simulink model "uz_mlp_three_layer"  (R2021a)
settings: Solver=FixedStepDiscrete  StartTime=0.0  StopTime=5000  RelTol=1e-3
values from neighbouring files (symbols this model uses):
  nn = nn.set_all_parameter(rand_variables)    [mlp2_definition.m]
  nn_data_type_max = 131071    [mlp2_definition.m]
  numInput = 13    [mlp2_definition.m]
  numOut = 4    [mlp2_definition.m]
libraries: hdlsllib x90, simulink x79, el_machinelearning x2
(part 1 of 4)
settings Model: DataTypeOverride=Off  Creator=ts  LastModifiedBy=ts
settings SolverCC: AlgebraicLoopSolver=TrustRegion
settings DataIOCC: SaveOutput=off  SaveTime=off
settings OptimizationCC: BlockReduction=off  ConditionallyExecuteInputs=off  DefaultParameterBehavior=Inlined
settings DebuggingCC: AlgebraicLoopMsg=error  SingleTaskRateTransMsg=error  SFMachineParentedDataDiag=warning
settings HardwareCC: ProdBitPerPointer=32  ProdBitPerSizeT=32  ProdBitPerPtrDiffT=32  ProdLargestAtomicFloat=None  ProdIntDivRoundTo=Undefined  ProdEndianess=Unspecified  ProdWordSize=32  ProdHWDeviceType=ASIC/FPGA->ASIC/FPGA  TargetBitPerLong=64  TargetBitPerPointer=64  TargetBitPerSizeT=64  TargetBitPerPtrDiffT=64  TargetLongLongMode=on  TargetIntDivRoundTo=Zero  TargetEndianess=LittleEndian  TargetWordSize=64  TargetHWDeviceType=Custom Processor->MATLAB Host Computer  ProdEqTarget=off

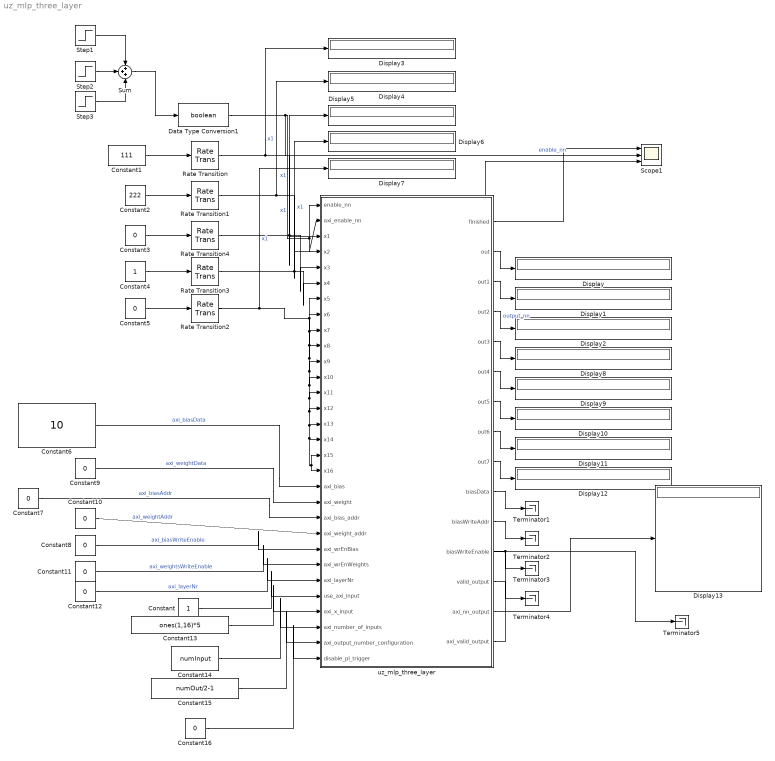
== system uz_mlp_three_layer ==
  Constant : Constant  OutDataTypeStr=boolean  SampleTime=-1
  Constant1 : Constant  Value=111  OutDataTypeStr=fixdt(1,32,14)
  Constant10 : Constant  Value=0  OutDataTypeStr=fixdt(0,10,0)  SampleTime=-1
  Constant11 : Constant  Value=0  OutDataTypeStr=uint8  SampleTime=-1
  Constant12 : Constant  Value=0  OutDataTypeStr=uint8  SampleTime=-1
  Constant13 : Constant  Value=ones(1,16)*5  OutDataTypeStr=fixdt(1,32,14)  SampleTime=-1
  Constant14 : Constant  Value=numInput  OutDataTypeStr=fixdt(0,10,0)  SampleTime=-1
  Constant15 : Constant  Value=numOut/2-1  OutDataTypeStr=fixdt(0,10,0)  SampleTime=-1
  Constant16 : Constant  Value=0  OutDataTypeStr=boolean  SampleTime=-1
  Constant2 : Constant  Value=222  OutDataTypeStr=fixdt(1,32,14)
  Constant3 : Constant  Value=0  OutDataTypeStr=fixdt(1,32,14)
  Constant4 : Constant  OutDataTypeStr=fixdt(1,32,14)
  Constant5 : Constant  Value=0  OutDataTypeStr=fixdt(1,32,14)
  Constant6 : Constant  Value=10  OutDataTypeStr=fixdt(1,32,14)  SampleTime=-1
  Constant7 : Constant  Value=0  OutDataTypeStr=fixdt(0,10,0)  SampleTime=-1
  Constant8 : Constant  Value=0  OutDataTypeStr=uint8  SampleTime=-1
  Constant9 : Constant  Value=0  OutDataTypeStr=fixdt(1,32,14)  SampleTime=-1
  Data Type Conversion1 : DataTypeConversion  OutDataTypeStr=boolean
  Display{,1..13} (14 alike) : Display
      Display11 settings: Format=hex (Stored Integer)
      Display3 settings: Format=hex (Stored Integer)
      Display4 settings: Format=hex (Stored Integer)
      Display5 settings: Format=hex (Stored Integer)
      Display6 settings: Format=hex (Stored Integer)
      Display7 settings: Format=hex (Stored Integer)
  Rate Transition{,1..4} (5 alike) : RateTransition
  Scope1 : Scope  NumInputPorts=3
  Step1 : Step  Time=2000  After=-1  SampleTime=1
  Step2 : Step  Time=100  SampleTime=1
  Step3 : Step  Time=2500  SampleTime=1
  Sum : Sum  Inputs=+++
  Terminator{1..5} (5 alike) : Terminator
  uz_mlp_three_layer : Subsystem  TreatAsAtomicUnit=on
  wires:
  Constant1/1 -> Rate Transition/1
  Constant5/1 -> Rate Transition2/1
  Constant2/1 -> Rate Transition1/1
  Constant3/1 -> Rate Transition4/1
  Constant4/1 -> Rate Transition3/1
  Data Type Conversion1/1 -> Scope1/2, uz_mlp_three_layer/2(axi_enable_nn), uz_mlp_three_layer/1(enable_nn)  "enable_nn"
  Rate Transition/1 -> uz_mlp_three_layer/3(x1), Display3/1  "x1"
  Rate Transition1/1 -> uz_mlp_three_layer/4(x2), Display4/1  "x1"
  Rate Transition4/1 -> Display5/1, uz_mlp_three_layer/5(x3)  "x1"
  Rate Transition3/1 -> Display6/1, uz_mlp_three_layer/6(x4)  "x1"
  Rate Transition2/1 -> uz_mlp_three_layer/8(x6), uz_mlp_three_layer/18(x16), uz_mlp_three_layer/17(x15), uz_mlp_three_layer/16(x14), uz_mlp_three_layer/15(x13), uz_mlp_three_layer/14(x12), uz_mlp_three_layer/13(x11), uz_mlp_three_layer/12(x10), uz_mlp_three_layer/11(x9), uz_mlp_three_layer/10(x8), uz_mlp_three_layer/9(x7), uz_mlp_three_layer/7(x5), Display7/1  "x1"
  uz_mlp_three_layer/2(out) -> Display/1
  uz_mlp_three_layer/3(out1) -> Display1/1
  uz_mlp_three_layer/4(out2) -> Display2/1  "output_nn"
  uz_mlp_three_layer/5(out3) -> Display8/1
  uz_mlp_three_layer/6(out4) -> Display9/1
  uz_mlp_three_layer/7(out5) -> Display10/1
  uz_mlp_three_layer/8(out6) -> Display11/1
  uz_mlp_three_layer/9(out7) -> Display12/1
  Constant6/1 -> uz_mlp_three_layer/19(axi_bias)  "axi_biasData"
  Constant7/1 -> uz_mlp_three_layer/21(axi_bias_addr)  "axi_biasAddr"
  Constant9/1 -> uz_mlp_three_layer/20(axi_weight)  "axi_weightData"
  Constant10/1 -> uz_mlp_three_layer/22(axi_weight_addr)  "axi_weightAddr"
  Constant8/1 -> uz_mlp_three_layer/23(axi_wrEnBias)  "axi_biasWriteEnable"
  Constant11/1 -> uz_mlp_three_layer/24(axi_wrEnWeights)  "axi_weightsWriteEnable"
  Constant12/1 -> uz_mlp_three_layer/25(axi_layerNr)  "axi_layerNr"
  uz_mlp_three_layer/10(biasData) -> Terminator1/1
  uz_mlp_three_layer/11(biasWriteAddr) -> Terminator2/1
  uz_mlp_three_layer/12(biasWriteEnable) -> Terminator3/1
  Step1/1 -> Sum/1
  Sum/1 -> Data Type Conversion1/1
  Step2/1 -> Sum/2
  Step3/1 -> Sum/3
  uz_mlp_three_layer/13(valid_output) -> Terminator4/1
  Constant/1 -> uz_mlp_three_layer/26(use_axi_input)
  Constant13/1 -> uz_mlp_three_layer/27(axi_x_input)
  uz_mlp_three_layer/14(axi_nn_output) -> Display13/1
  uz_mlp_three_layer/15(axi_valid_output) -> Scope1/3, Terminator5/1
  Constant14/1 -> uz_mlp_three_layer/28(axi_number_of_inputs)
  Constant15/1 -> uz_mlp_three_layer/29(axi_output_number_configuration)
  uz_mlp_three_layer/1(finished) -> Scope1/1
  Constant16/1 -> uz_mlp_three_layer/30(disable_pl_trigger)

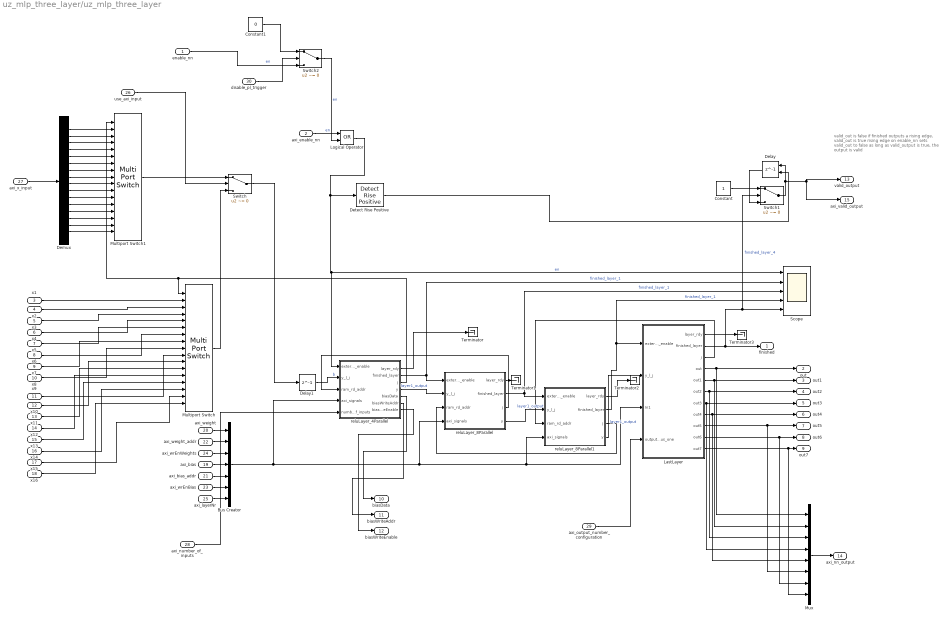
== system uz_mlp_three_layer/uz_mlp_three_layer ==
  note: valid_out is false
      | if finished outputs a rising edge, valid_out is true
      | rising edge on enable_nn sets valid_out to false
      |
      | as long as valid_output is true, the output is valid
  enable_nn : Inport
  axi_enable_nn : Inport  Port=2
  x1 : Inport  Port=3
  x2 : Inport  Port=4
  x3 : Inport  Port=5
  x4 : Inport  Port=6
  x5 : Inport  Port=7
  x6 : Inport  Port=8
  x7 : Inport  Port=9
  x8 : Inport  Port=10
  x9 : Inport  Port=11
  x10 : Inport  Port=12
  x11 : Inport  Port=13
  x12 : Inport  Port=14
  x13 : Inport  Port=15
  x14 : Inport  Port=16
  x15 : Inport  Port=17
  x16 : Inport  Port=18
  axi_bias : Inport  Port=19
  axi_weight : Inport  Port=20
  axi_bias_addr : Inport  Port=21
  axi_weight_addr : Inport  Port=22
  axi_wrEnBias : Inport  Port=23
  axi_wrEnWeights : Inport  Port=24
  axi_layerNr : Inport  Port=25
  use_axi_input : Inport  Port=26
  axi_x_input : Inport  Port=27
  axi_number_of_inputs : Inport  Port=28
  axi_output_number_configuration : Inport  Port=29
  disable_pl_trigger : Inport  Port=30
  Bus Creator : BusCreator  Inputs=7
  Constant : Constant  OutDataTypeStr=boolean  SampleTime=-1
  Constant1 : Constant  Value=0  OutDataTypeStr=boolean  SampleTime=-1
  Delay : Delay  DelayLength=1  ExternalReset=Level
      settings: InputPortMap=u0,r5
  Delay1 : Delay  DelayLength=1
  Demux : Demux  Outputs=16
  Detect Rise Positive : simulink/Logic and Bit Operations/Detect Rise Positive  vinit=0  OutDataTypeStr=boolean
  LastLayer : Subsystem  TreatAsAtomicUnit=on  mask{layer=nn.layer(4), ParallelDSP=2, nNeurons=numOut, LayerNr=4}
      mask prompts: layer "Layer number:"; ParallelDSP "Number of parallel DSP"; nNeurons "Number of neurons in layer"; LayerNr "Number of this Layer"
  Logical Operator : Logic  Operator=OR  AllPortsSameDT=off  OutDataTypeStr=boolean
  Multiport Switch : MultiPortSwitch  Inputs=16
  Multiport Switch1 : MultiPortSwitch  Inputs=16
  Mux : Mux  Inputs=8
  Scope : Scope  NumInputPorts=5
  Switch : Switch  Criteria=u2 ~= 0
  Switch1 : Switch  Criteria=u2 ~= 0
  Switch2 : Switch  Criteria=u2 ~= 0
  Terminator{,1..3} (4 alike) : Terminator
  reluLayer_4Parallel : Subsystem  TreatAsAtomicUnit=on  mask{layer=nn.layer(1), ParallelDSP=4, nNeurons=64, LayerNr=1}
      mask prompts: layer "Layer data"; ParallelDSP "Number of parallel DSP"; nNeurons "Number of neurons in layer"; LayerNr "Number of this layer"
  reluLayer_8Parallel : Subsystem  TreatAsAtomicUnit=on  mask{layer=nn.layer(2), LayerNr=2, ParallelDSP=8, nNeurons=64}
      mask prompts: layer "Layer data"; LayerNr "Number of this layer"; ParallelDSP "Number of parallel DSP"; nNeurons "Number of neurons in layer"
  reluLayer_8Parallel1 : Subsystem  TreatAsAtomicUnit=on  mask{layer=nn.layer(3), LayerNr=3, ParallelDSP=8, nNeurons=64}
      mask prompts: layer "Layer data"; LayerNr "Number of this layer"; ParallelDSP "Number of parallel DSP"; nNeurons "Number of neurons in layer"
  finished : Outport
  out : Outport  Port=2
  out1 : Outport  Port=3
  out2 : Outport  Port=4
  out3 : Outport  Port=5
  out4 : Outport  Port=6
  out5 : Outport  Port=7
  out6 : Outport  Port=8
  out7 : Outport  Port=9
  biasData : Outport  Port=10
  biasWriteAddr : Outport  Port=11
  biasWriteEnable : Outport  Port=12
  valid_output : Outport  Port=13
  axi_nn_output : Outport  Port=14
  axi_valid_output : Outport  Port=15
  wires:
  Logical Operator/1 -> reluLayer_4Parallel/1(external_enable), Scope/1, Detect Rise Positive/1  "en"
  x2/1 -> Multiport Switch/3
  reluLayer_4Parallel/3(j) -> Multiport Switch/1, Multiport Switch1/1
  x4/1 -> Multiport Switch/5
  x5/1 -> Multiport Switch/6
  x1/1 -> Multiport Switch/2
  Delay1/1 -> reluLayer_4Parallel/2(y_l_j)  "b"
  x3/1 -> Multiport Switch/4
  LastLayer/2(finished_layer) -> finished/1, Switch1/2, Scope/5  "finished_layer_4"
  reluLayer_4Parallel/2(finished_layer) -> reluLayer_8Parallel/1(external_enable), Scope/2  "finished_layer_1"
  reluLayer_8Parallel1/4(y) -> LastLayer/2(y_l_j)  "layer1_output"
  reluLayer_8Parallel/2(finished_layer) -> reluLayer_8Parallel1/1(external_enable), Scope/3  "finished_layer_1"
  reluLayer_8Parallel/4(y) -> reluLayer_8Parallel1/2(y_l_j)  "layer1_output"
  reluLayer_8Parallel1/2(finished_layer) -> Scope/4, LastLayer/1(external_enable)  "finished_layer_1"
  LastLayer/4(out) -> Mux/1, out/1
  LastLayer/5(out1) -> Mux/2, out1/1
  LastLayer/6(out2) -> Mux/3, out2/1
  LastLayer/7(out3) -> Mux/4, out3/1
  LastLayer/8(out4) -> Mux/5, out4/1
  LastLayer/9(out5) -> Mux/6, out5/1
  LastLayer/10(out6) -> Mux/7, out6/1
  LastLayer/11(out7) -> Mux/8, out7/1
  Bus Creator/1 -> reluLayer_4Parallel/4(axi_signals), reluLayer_8Parallel/4(axi_signals), reluLayer_8Parallel1/4(axi_signals), LastLayer/3(In1)
  axi_weight/1 -> Bus Creator/1
  axi_weight_addr/1 -> Bus Creator/2
  axi_wrEnWeights/1 -> Bus Creator/3
  axi_bias/1 -> Bus Creator/4
  axi_bias_addr/1 -> Bus Creator/5
  axi_wrEnBias/1 -> Bus Creator/6
  reluLayer_8Parallel/3(j) -> reluLayer_4Parallel/3(ram_rd_addr)
  axi_layerNr/1 -> Bus Creator/7
  reluLayer_8Parallel1/3(j) -> reluLayer_8Parallel/3(ram_rd_addr)
  LastLayer/3(j) -> reluLayer_8Parallel1/3(ram_rd_addr)
  reluLayer_4Parallel/1(layer_rdy) -> Terminator/1
  reluLayer_8Parallel/1(layer_rdy) -> Terminator1/1
  reluLayer_8Parallel1/1(layer_rdy) -> Terminator2/1
  reluLayer_4Parallel/5(biasData) -> biasData/1
  reluLayer_4Parallel/6(biasWriteAddr) -> biasWriteAddr/1
  reluLayer_4Parallel/7(biasWriteEnable) -> biasWriteEnable/1
  reluLayer_4Parallel/4(y) -> reluLayer_8Parallel/2(y_l_j)  "layer1_output"
  Detect Rise Positive/1 -> Delay/2
  Switch1/1 -> valid_output/1, axi_valid_output/1, Delay/1
  x6/1 -> Multiport Switch/7
  x7/1 -> Multiport Switch/8
  x8/1 -> Multiport Switch/9
  x9/1 -> Multiport Switch/10
  x10/1 -> Multiport Switch/11
  x11/1 -> Multiport Switch/12
  x12/1 -> Multiport Switch/13
  x13/1 -> Multiport Switch/14
  x14/1 -> Multiport Switch/15
  x15/1 -> Multiport Switch/16
  x16/1 -> Multiport Switch/17
  Demux/1 -> Multiport Switch1/2
  Demux/2 -> Multiport Switch1/3
  Demux/3 -> Multiport Switch1/4
  Demux/4 -> Multiport Switch1/5
  Demux/5 -> Multiport Switch1/6
  Demux/6 -> Multiport Switch1/7
  Demux/7 -> Multiport Switch1/8
  Demux/8 -> Multiport Switch1/9
  Demux/9 -> Multiport Switch1/10
  Demux/10 -> Multiport Switch1/11
  Demux/11 -> Multiport Switch1/12
  Demux/12 -> Multiport Switch1/13
  Demux/13 -> Multiport Switch1/14
  Demux/14 -> Multiport Switch1/15
  Demux/15 -> Multiport Switch1/16
  Demux/16 -> Multiport Switch1/17
  Switch/1 -> Delay1/1
  Multiport Switch/1 -> Switch/3
  Multiport Switch1/1 -> Switch/1
  use_axi_input/1 -> Switch/2
  axi_x_input/1 -> Demux/1
  Mux/1 -> axi_nn_output/1
  Delay/1 -> Switch1/3
  Constant/1 -> Switch1/1
  axi_number_of_inputs/1 -> reluLayer_4Parallel/5(number_of_inputs)
  axi_output_number_configuration/1 -> LastLayer/4(output_half_minus_one)
  axi_enable_nn/1 -> Logical Operator/1  "en"
  Switch2/1 -> Logical Operator/2  "en"
  LastLayer/1(layer_rdy) -> Terminator3/1
  enable_nn/1 -> Switch2/3  "en"
  disable_pl_trigger/1 -> Switch2/2
  Constant1/1 -> Switch2/1

== system uz_mlp_three_layer/uz_mlp_three_layer/LastLayer ==
  external_enable : Inport
  y_l_j : Inport  Port=2
  In1 : Inport  Port=3
  output_half_minus_one : Inport  Port=4
  StateMachines : Subsystem
  Subsystem1 : Subsystem  mask{nStart=(1-1)*(nNeurons/ParallelDSP)+1, nEnd=(1-1)*(nNeurons/ParallelDSP)+(nNeurons/ParallelDSP), ParallelNr=1}
      mask prompts: nStart "First neuron (p=nr. of parallel MAC)"; nEnd "Last neuron"; ParallelNr "Nr of Parallel PCU"
  Subsystem8 : Subsystem  mask{nStart=(2-1)*(nNeurons/ParallelDSP)+1, nEnd=(2-1)*(nNeurons/ParallelDSP)+(nNeurons/ParallelDSP), ParallelNr=2}
      mask prompts: nStart "First neuron (p=nr. of parallel MAC)"; nEnd "Last neuron"; ParallelNr "Nr of Parallel PCU"
  Terminator : Terminator
  Terminator1 : Terminator
  parallelOutput : Subsystem
  layer_rdy : Outport
  finished_layer : Outport  Port=2
  j : Outport  Port=3
  out : Outport  Port=4
  out1 : Outport  Port=5
  out2 : Outport  Port=6
  out3 : Outport  Port=7
  out4 : Outport  Port=8
  out5 : Outport  Port=9
  out6 : Outport  Port=10
  out7 : Outport  Port=11
  wires:
  y_l_j/1 -> Subsystem1/2(b), Subsystem8/2(b)  "b"
  StateMachines/7(layer_rdy) -> layer_rdy/1
  parallelOutput/2(out1) -> out1/1
  StateMachines/4(startin) -> Subsystem1/3(startin), Subsystem8/3(startin)
  parallelOutput/3(out2) -> out2/1
  parallelOutput/6(out5) -> out5/1
  parallelOutput/8(out7) -> out7/1
  Subsystem1/1(rd_dout) -> parallelOutput/1(data_Upper)
  StateMachines/2(write_enable) -> parallelOutput/3(write_enable)
  StateMachines/5(endin) -> Subsystem1/4(endin), Subsystem8/4(endin)
  Subsystem1/2(startOut) -> StateMachines/2(mac_startOut)
  parallelOutput/7(out6) -> out6/1
  parallelOutput/4(out3) -> out3/1
  StateMachines/3(mac_counter) -> j/1, Subsystem8/1(mac_counter), Subsystem1/1(mac_counter)
  parallelOutput/1(out) -> out/1
  StateMachines/6(validIn) -> Subsystem1/5(validIn), Subsystem8/5(validIn)
  parallelOutput/5(out4) -> out4/1
  Subsystem1/3(endOut) -> StateMachines/1(end_out)
  StateMachines/1(n_perceptron) -> Subsystem1/6(n_perceptron), Subsystem8/6(n_perceptron), parallelOutput/2(n_perceptron)
  StateMachines/8(layer_finished) -> finished_layer/1
  external_enable/1 -> StateMachines/3(U)
  Subsystem8/1(rd_dout) -> parallelOutput/4(data_lower)
  In1/1 -> Subsystem8/7(axi_signals), Subsystem1/7(axi_signals)
  Subsystem8/2(startOut) -> Terminator/1
  Subsystem8/3(endOut) -> Terminator1/1
  output_half_minus_one/1 -> StateMachines/4(output_half_minus_one)

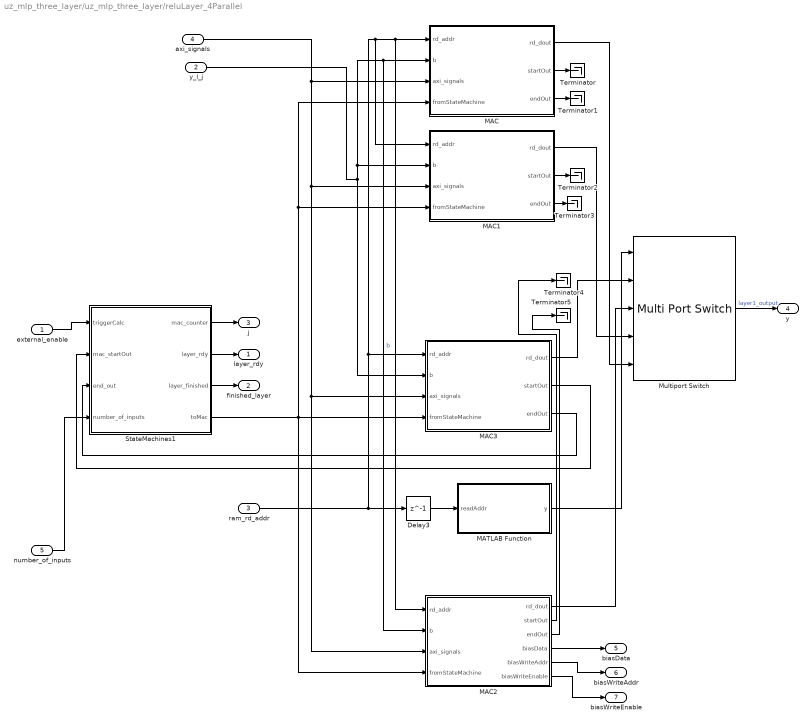
== system uz_mlp_three_layer/uz_mlp_three_layer/reluLayer_4Parallel ==
  external_enable : Inport
  y_l_j : Inport  Port=2
  ram_rd_addr : Inport  Port=3
  axi_signals : Inport  Port=4
  number_of_inputs : Inport  Port=5
  Delay3 : Delay  DelayLength=1
  MAC : Subsystem  AncestorBlock=el_machinelearning/neuralNetwork/MAC  mask{nStart=(4-1)*(nNeurons/ParallelDSP)+1, nEnd=(4-1)*(nNeurons/ParallelDSP)+(nNeurons/ParallelDSP), ParallelNr=4}
      mask prompts: nStart "First neuron (p=nr. of parallel MAC)"; nEnd "Last neuron"; ParallelNr "Nr of Parallel PCU"
  MAC1 : Subsystem  AncestorBlock=el_machinelearning/neuralNetwork/MAC  mask{nStart=(3-1)*(nNeurons/ParallelDSP)+1, nEnd=(3-1)*(nNeurons/ParallelDSP)+(nNeurons/ParallelDSP), ParallelNr=3}
      mask prompts: nStart "First neuron (p=nr. of parallel MAC)"; nEnd "Last neuron"; ParallelNr "Nr of Parallel PCU"
  MAC2 : Subsystem  AncestorBlock=el_machinelearning/neuralNetwork/MAC  mask{nStart=(2-1)*(nNeurons/ParallelDSP)+1, nEnd=(2-1)*(nNeurons/ParallelDSP)+(nNeurons/ParallelDSP), ParallelNr=2}
      mask prompts: nStart "First neuron (p=nr. of parallel MAC)"; nEnd "Last neuron"; ParallelNr "Nr of Parallel PCU"
  MAC3 : Subsystem  AncestorBlock=el_machinelearning/neuralNetwork/MAC  mask{nStart=(1-1)*(nNeurons/ParallelDSP)+1, nEnd=(1-1)*(nNeurons/ParallelDSP)+(nNeurons/ParallelDSP), ParallelNr=1}
      mask prompts: nStart "First neuron (p=nr. of parallel MAC)"; nEnd "Last neuron"; ParallelNr "Nr of Parallel PCU"
  MATLAB Function : MATLAB Function  TreatAsAtomicUnit=on
  Multiport Switch : MultiPortSwitch  DataPortOrder=Zero-based contiguous  Inputs=ParallelDSP  DataPortIndices={[0:16],[17:32],[33:48],[49:64]}  zeroidx=on
  StateMachines1 : Subsystem  AncestorBlock=el_machinelearning/neuralNetwork/StateMachines
  Terminator{,1..5} (6 alike) : Terminator
  layer_rdy : Outport
  finished_layer : Outport  Port=2
  j : Outport  Port=3
  y : Outport  Port=4
  biasData : Outport  Port=5
  biasWriteAddr : Outport  Port=6
  biasWriteEnable : Outport  Port=7
  wires:
  y_l_j/1 -> MAC3/2(b), MAC1/2(b), MAC2/2(b), MAC/2(b)  "b"
  ram_rd_addr/1 -> Delay3/1, MAC3/1(rd_addr), MAC1/1(rd_addr), MAC/1(rd_addr), MAC2/1(rd_addr)
  StateMachines1/2(layer_rdy) -> layer_rdy/1
  external_enable/1 -> StateMachines1/1(triggerCalc)
  MAC3/3(endOut) -> StateMachines1/3(end_out)
  MAC3/2(startOut) -> StateMachines1/2(mac_startOut)
  StateMachines1/3(layer_finished) -> finished_layer/1
  StateMachines1/1(mac_counter) -> j/1
  MAC2/1(rd_dout) -> Multiport Switch/3
  MAC3/1(rd_dout) -> Multiport Switch/2
  Multiport Switch/1 -> y/1  "layer1_output"
  Delay3/1 -> MATLAB Function/1(readAddr)
  MAC1/1(rd_dout) -> Multiport Switch/4
  MAC/1(rd_dout) -> Multiport Switch/5
  MATLAB Function/1(y) -> Multiport Switch/1
  axi_signals/1 -> MAC/3(axi_signals), MAC1/3(axi_signals), MAC3/3(axi_signals), MAC2/3(axi_signals)
  StateMachines1/4(toMac) -> MAC1/4(fromStateMachine), MAC/4(fromStateMachine), MAC2/4(fromStateMachine), MAC3/4(fromStateMachine)
  MAC/2(startOut) -> Terminator/1
  MAC/3(endOut) -> Terminator1/1
  MAC1/2(startOut) -> Terminator2/1
  MAC1/3(endOut) -> Terminator3/1
  MAC2/2(startOut) -> Terminator4/1
  MAC2/3(endOut) -> Terminator5/1
  MAC2/4(biasData) -> biasData/1
  MAC2/5(biasWriteAddr) -> biasWriteAddr/1
  MAC2/6(biasWriteEnable) -> biasWriteEnable/1
  number_of_inputs/1 -> StateMachines1/4(number_of_inputs)

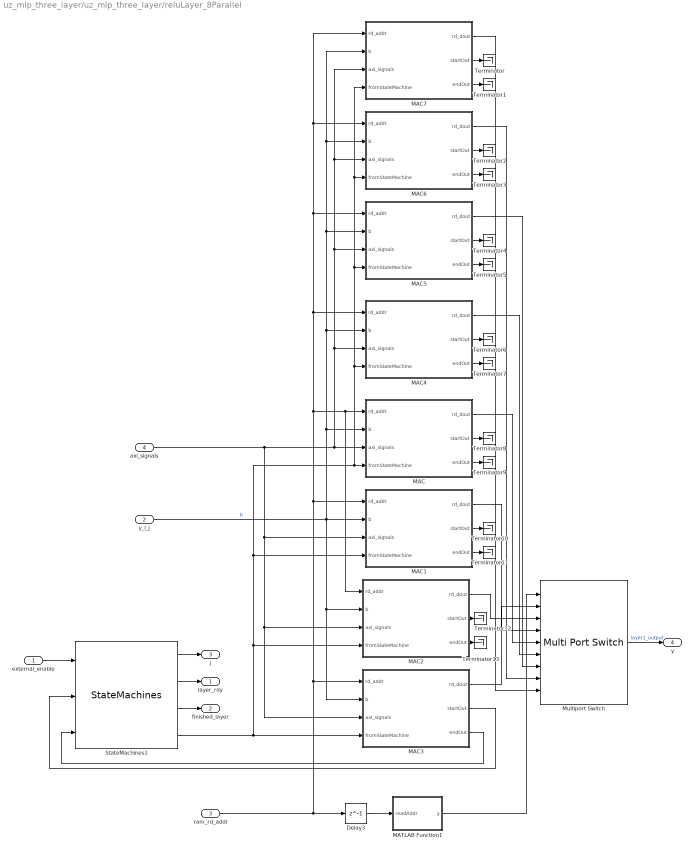
== system uz_mlp_three_layer/uz_mlp_three_layer/reluLayer_8Parallel ==
  external_enable : Inport
  y_l_j : Inport  Port=2
  ram_rd_addr : Inport  Port=3
  axi_signals : Inport  Port=4
  Delay3 : Delay  DelayLength=1
  MAC : Subsystem  AncestorBlock=el_machinelearning/neuralNetwork/MAC  mask{nStart=(4-1)*(nNeurons/ParallelDSP)+1, nEnd=(4-1)*(nNeurons/ParallelDSP)+(nNeurons/ParallelDSP), ParallelNr=4}
      mask prompts: nStart "First neuron (p=nr. of parallel MAC)"; nEnd "Last neuron"; ParallelNr "Nr of Parallel PCU"
  MAC1 : Subsystem  AncestorBlock=el_machinelearning/neuralNetwork/MAC  mask{nStart=(3-1)*(nNeurons/ParallelDSP)+1, nEnd=(3-1)*(nNeurons/ParallelDSP)+(nNeurons/ParallelDSP), ParallelNr=3}
      mask prompts: nStart "First neuron (p=nr. of parallel MAC)"; nEnd "Last neuron"; ParallelNr "Nr of Parallel PCU"
  MAC2 : Subsystem  AncestorBlock=el_machinelearning/neuralNetwork/MAC  mask{nStart=(2-1)*(nNeurons/ParallelDSP)+1, nEnd=(2-1)*(nNeurons/ParallelDSP)+(nNeurons/ParallelDSP), ParallelNr=2}
      mask prompts: nStart "First neuron (p=nr. of parallel MAC)"; nEnd "Last neuron"; ParallelNr "Nr of Parallel PCU"
  MAC3 : Subsystem  AncestorBlock=el_machinelearning/neuralNetwork/MAC  mask{nStart=(1-1)*(nNeurons/ParallelDSP)+1, nEnd=(1-1)*(nNeurons/ParallelDSP)+(nNeurons/ParallelDSP), ParallelNr=1}
      mask prompts: nStart "First neuron (p=nr. of parallel MAC)"; nEnd "Last neuron"; ParallelNr "Nr of Parallel PCU"
  MAC4 : Subsystem  AncestorBlock=el_machinelearning/neuralNetwork/MAC  mask{nStart=(5-1)*(nNeurons/ParallelDSP)+1, nEnd=(5-1)*(nNeurons/ParallelDSP)+(nNeurons/ParallelDSP), ParallelNr=5}
      mask prompts: nStart "First neuron (p=nr. of parallel MAC)"; nEnd "Last neuron"; ParallelNr "Nr of Parallel PCU"
  MAC5 : Subsystem  AncestorBlock=el_machinelearning/neuralNetwork/MAC  mask{nStart=(6-1)*(nNeurons/ParallelDSP)+1, nEnd=(6-1)*(nNeurons/ParallelDSP)+(nNeurons/ParallelDSP), ParallelNr=6}
      mask prompts: nStart "First neuron (p=nr. of parallel MAC)"; nEnd "Last neuron"; ParallelNr "Nr of Parallel PCU"
  MAC6 : Subsystem  AncestorBlock=el_machinelearning/neuralNetwork/MAC  mask{nStart=(7-1)*(nNeurons/ParallelDSP)+1, nEnd=(7-1)*(nNeurons/ParallelDSP)+(nNeurons/ParallelDSP), ParallelNr=7}
      mask prompts: nStart "First neuron (p=nr. of parallel MAC)"; nEnd "Last neuron"; ParallelNr "Nr of Parallel PCU"
  MAC7 : Subsystem  AncestorBlock=el_machinelearning/neuralNetwork/MAC  mask{nStart=(8-1)*(nNeurons/ParallelDSP)+1, nEnd=(8-1)*(nNeurons/ParallelDSP)+(nNeurons/ParallelDSP), ParallelNr=8}
      mask prompts: nStart "First neuron (p=nr. of parallel MAC)"; nEnd "Last neuron"; ParallelNr "Nr of Parallel PCU"
  MATLAB Function1 : MATLAB Function  TreatAsAtomicUnit=on
  Multiport Switch : MultiPortSwitch  DataPortOrder=Zero-based contiguous  Inputs=ParallelDSP  DataPortIndices={[0:16],[17:32],[33:48],[49:64]}  zeroidx=on
  StateMachines1 : el_machinelearning/neuralNetwork/StateMachines  SystemSampleTime=-1  VariantActivationTime=update diagram  Latency=0  AutoFrameSizeCalculation=off
  Terminator{,1..13} (14 alike) : Terminator
  layer_rdy : Outport
  finished_layer : Outport  Port=2
  j : Outport  Port=3
  y : Outport  Port=4
  wires:
  y_l_j/1 -> MAC2/2(b), MAC3/2(b), MAC1/2(b), MAC7/2(b), MAC6/2(b), MAC5/2(b), MAC4/2(b), MAC/2(b)  "b"
  ram_rd_addr/1 -> Delay3/1, MAC3/1(rd_addr), MAC7/1(rd_addr), MAC6/1(rd_addr), MAC5/1(rd_addr), MAC4/1(rd_addr), MAC2/1(rd_addr), MAC/1(rd_addr), MAC1/1(rd_addr)
  StateMachines1/2 -> layer_rdy/1
  external_enable/1 -> StateMachines1/1
  MAC3/3(endOut) -> StateMachines1/3
  MAC3/2(startOut) -> StateMachines1/2
  StateMachines1/3 -> finished_layer/1
  StateMachines1/1 -> j/1
  MAC2/1(rd_dout) -> Multiport Switch/3
  MAC3/1(rd_dout) -> Multiport Switch/2
  Multiport Switch/1 -> y/1  "layer1_output"
  Delay3/1 -> MATLAB Function1/1(readAddr)
  MAC1/1(rd_dout) -> Multiport Switch/4
  MAC/1(rd_dout) -> Multiport Switch/5
  MATLAB Function1/1(y) -> Multiport Switch/1
  axi_signals/1 -> MAC7/3(axi_signals), MAC6/3(axi_signals), MAC5/3(axi_signals), MAC4/3(axi_signals), MAC/3(axi_signals), MAC2/3(axi_signals), MAC3/3(axi_signals), MAC1/3(axi_signals)
  StateMachines1/4 -> MAC3/4(fromStateMachine), MAC2/4(fromStateMachine), MAC7/4(fromStateMachine), MAC6/4(fromStateMachine), MAC5/4(fromStateMachine), MAC4/4(fromStateMachine), MAC/4(fromStateMachine), MAC1/4(fromStateMachine)
  MAC4/1(rd_dout) -> Multiport Switch/6
  MAC5/1(rd_dout) -> Multiport Switch/7
  MAC6/1(rd_dout) -> Multiport Switch/8
  MAC7/1(rd_dout) -> Multiport Switch/9
  MAC7/2(startOut) -> Terminator/1
  MAC7/3(endOut) -> Terminator1/1
  MAC6/2(startOut) -> Terminator2/1
  MAC6/3(endOut) -> Terminator3/1
  MAC5/2(startOut) -> Terminator4/1
  MAC5/3(endOut) -> Terminator5/1
  MAC4/2(startOut) -> Terminator6/1
  MAC4/3(endOut) -> Terminator7/1
  MAC/2(startOut) -> Terminator8/1
  MAC/3(endOut) -> Terminator9/1
  MAC1/2(startOut) -> Terminator10/1
  MAC1/3(endOut) -> Terminator11/1
  MAC2/2(startOut) -> Terminator12/1
  MAC2/3(endOut) -> Terminator13/1

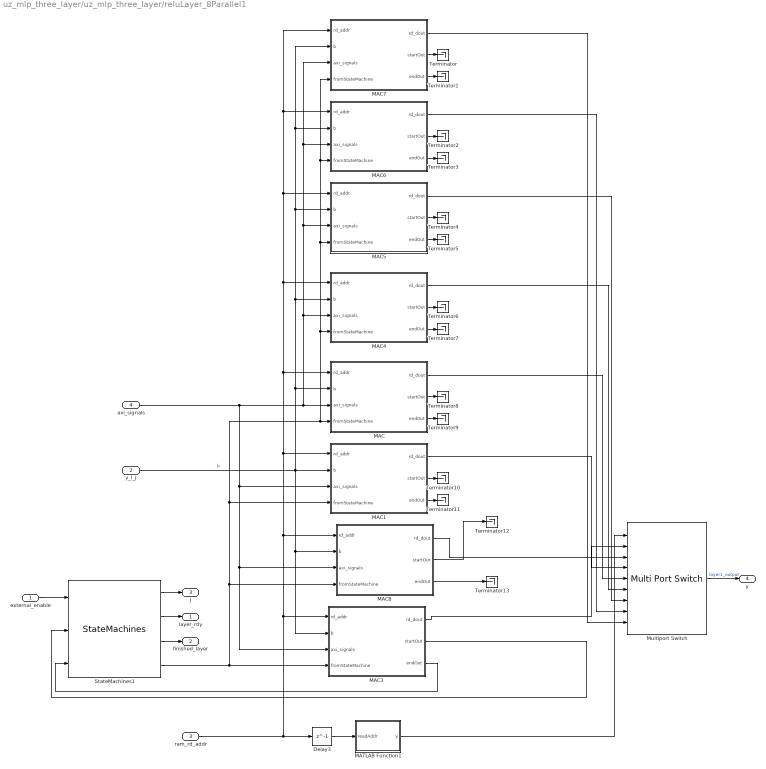
== system uz_mlp_three_layer/uz_mlp_three_layer/reluLayer_8Parallel1 ==
  external_enable : Inport
  y_l_j : Inport  Port=2
  ram_rd_addr : Inport  Port=3
  axi_signals : Inport  Port=4
  Delay3 : Delay  DelayLength=1
  MAC : Subsystem  AncestorBlock=el_machinelearning/neuralNetwork/MAC  mask{nStart=(4-1)*(nNeurons/ParallelDSP)+1, nEnd=(4-1)*(nNeurons/ParallelDSP)+(nNeurons/ParallelDSP), ParallelNr=4}
      mask prompts: nStart "First neuron (p=nr. of parallel MAC)"; nEnd "Last neuron"; ParallelNr "Nr of Parallel PCU"
  MAC1 : Subsystem  AncestorBlock=el_machinelearning/neuralNetwork/MAC  mask{nStart=(3-1)*(nNeurons/ParallelDSP)+1, nEnd=(3-1)*(nNeurons/ParallelDSP)+(nNeurons/ParallelDSP), ParallelNr=3}
      mask prompts: nStart "First neuron (p=nr. of parallel MAC)"; nEnd "Last neuron"; ParallelNr "Nr of Parallel PCU"
  MAC3 : Subsystem  AncestorBlock=el_machinelearning/neuralNetwork/MAC  mask{nStart=(1-1)*(nNeurons/ParallelDSP)+1, nEnd=(1-1)*(nNeurons/ParallelDSP)+(nNeurons/ParallelDSP), ParallelNr=1}
      mask prompts: nStart "First neuron (p=nr. of parallel MAC)"; nEnd "Last neuron"; ParallelNr "Nr of Parallel PCU"
  MAC4 : Subsystem  AncestorBlock=el_machinelearning/neuralNetwork/MAC  mask{nStart=(5-1)*(nNeurons/ParallelDSP)+1, nEnd=(5-1)*(nNeurons/ParallelDSP)+(nNeurons/ParallelDSP), ParallelNr=5}
      mask prompts: nStart "First neuron (p=nr. of parallel MAC)"; nEnd "Last neuron"; ParallelNr "Nr of Parallel PCU"
  MAC5 : Subsystem  AncestorBlock=el_machinelearning/neuralNetwork/MAC  mask{nStart=(6-1)*(nNeurons/ParallelDSP)+1, nEnd=(6-1)*(nNeurons/ParallelDSP)+(nNeurons/ParallelDSP), ParallelNr=6}
      mask prompts: nStart "First neuron (p=nr. of parallel MAC)"; nEnd "Last neuron"; ParallelNr "Nr of Parallel PCU"
  MAC6 : Subsystem  AncestorBlock=el_machinelearning/neuralNetwork/MAC  mask{nStart=(7-1)*(nNeurons/ParallelDSP)+1, nEnd=(7-1)*(nNeurons/ParallelDSP)+(nNeurons/ParallelDSP), ParallelNr=7}
      mask prompts: nStart "First neuron (p=nr. of parallel MAC)"; nEnd "Last neuron"; ParallelNr "Nr of Parallel PCU"
  MAC7 : Subsystem  AncestorBlock=el_machinelearning/neuralNetwork/MAC  mask{nStart=(8-1)*(nNeurons/ParallelDSP)+1, nEnd=(8-1)*(nNeurons/ParallelDSP)+(nNeurons/ParallelDSP), ParallelNr=8}
      mask prompts: nStart "First neuron (p=nr. of parallel MAC)"; nEnd "Last neuron"; ParallelNr "Nr of Parallel PCU"
  MAC8 : Subsystem  AncestorBlock=el_machinelearning/neuralNetwork/MAC  mask{nStart=(2-1)*(nNeurons/ParallelDSP)+1, nEnd=(2-1)*(nNeurons/ParallelDSP)+(nNeurons/ParallelDSP), ParallelNr=2}
      mask prompts: nStart "First neuron (p=nr. of parallel MAC)"; nEnd "Last neuron"; ParallelNr "Nr of Parallel PCU"
  MATLAB Function1 : MATLAB Function  TreatAsAtomicUnit=on
  Multiport Switch : MultiPortSwitch  DataPortOrder=Zero-based contiguous  Inputs=ParallelDSP  DataPortIndices={[0:16],[17:32],[33:48],[49:64]}  zeroidx=on
  StateMachines1 : el_machinelearning/neuralNetwork/StateMachines  SystemSampleTime=-1  VariantActivationTime=update diagram  Latency=0  AutoFrameSizeCalculation=off
  Terminator{,1..13} (14 alike) : Terminator
  layer_rdy : Outport
  finished_layer : Outport  Port=2
  j : Outport  Port=3
  y : Outport  Port=4
  wires:
  MAC8/3(endOut) -> Terminator13/1
  MAC8/2(startOut) -> Terminator12/1
  MAC1/3(endOut) -> Terminator11/1
  MAC1/2(startOut) -> Terminator10/1
  MAC/3(endOut) -> Terminator9/1
  MAC/2(startOut) -> Terminator8/1
  MAC4/3(endOut) -> Terminator7/1
  MAC4/2(startOut) -> Terminator6/1
  MAC5/3(endOut) -> Terminator5/1
  MAC5/2(startOut) -> Terminator4/1
  MAC6/3(endOut) -> Terminator3/1
  MAC6/2(startOut) -> Terminator2/1
  MAC7/3(endOut) -> Terminator1/1
  MAC7/2(startOut) -> Terminator/1
  MAC7/1(rd_dout) -> Multiport Switch/9
  MAC6/1(rd_dout) -> Multiport Switch/8
  MAC5/1(rd_dout) -> Multiport Switch/7
  MAC4/1(rd_dout) -> Multiport Switch/6
  StateMachines1/4 -> MAC8/4(fromStateMachine), MAC1/4(fromStateMachine), MAC/4(fromStateMachine), MAC4/4(fromStateMachine), MAC5/4(fromStateMachine), MAC6/4(fromStateMachine), MAC7/4(fromStateMachine), MAC3/4(fromStateMachine)
  axi_signals/1 -> MAC1/3(axi_signals), MAC3/3(axi_signals), MAC8/3(axi_signals), MAC/3(axi_signals), MAC4/3(axi_signals), MAC5/3(axi_signals), MAC6/3(axi_signals), MAC7/3(axi_signals)
  MATLAB Function1/1(y) -> Multiport Switch/1
  MAC/1(rd_dout) -> Multiport Switch/5
  MAC1/1(rd_dout) -> Multiport Switch/4
  Delay3/1 -> MATLAB Function1/1(readAddr)
  Multiport Switch/1 -> y/1  "layer1_output"
  MAC3/1(rd_dout) -> Multiport Switch/2
  MAC8/1(rd_dout) -> Multiport Switch/3
  StateMachines1/1 -> j/1
  StateMachines1/3 -> finished_layer/1
  MAC3/2(startOut) -> StateMachines1/2
  MAC3/3(endOut) -> StateMachines1/3
  external_enable/1 -> StateMachines1/1
  StateMachines1/2 -> layer_rdy/1
  ram_rd_addr/1 -> MAC/1(rd_addr), MAC4/1(rd_addr), MAC5/1(rd_addr), MAC6/1(rd_addr), MAC7/1(rd_addr), MAC1/1(rd_addr), MAC8/1(rd_addr), MAC3/1(rd_addr), Delay3/1
  y_l_j/1 -> MAC/2(b), MAC4/2(b), MAC5/2(b), MAC6/2(b), MAC7/2(b), MAC1/2(b), MAC3/2(b), MAC8/2(b)  "b"

== system uz_mlp_three_layer/uz_mlp_three_layer/LastLayer/StateMachines ==
  end_out : Inport
  mac_startOut : Inport  Port=2
  U : Inport  Port=3
  output_half_minus_one : Inport  Port=4
  Compare To Constant : simulink/Logic and Bit Operations/Compare To Constant  relop===  const=layer.weight_dimension(1)  OutDataTypeStr=boolean
  Delay2 : Delay  DelayLength=1
  Delay3 : Delay  DelayLength=1
  Delay4 : Delay  DelayLength=1
  Detect Rise Positive : simulink/Logic and Bit Operations/Detect Rise Positive  vinit=0  OutDataTypeStr=boolean
  Relational Operator : RelationalOperator  Operator===  OutDataTypeStr=boolean  RndMeth=Simplest
  Scope : Scope  NumInputPorts=2
  index_counter : hdlsllib/Sources/HDL Counter  CountType=Count limited  CountInit=1  CountStep=1  CountMax=layer.weight_dimension(1)  CountFromType=Initial value  CountFrom=1  CountResetPort=on  CountLoadPort=off  CountEnbPort=on  CountDirPort=off  CountHitOutputPort=off  CountDataType=Unsigned  CountWordLen=10  CountFracLen=0  CountSampTime=1
  layer_control : Stateflow chart  TreatAsAtomicUnit=on
  mac_control : Stateflow chart  TreatAsAtomicUnit=on
  perceptron_counter1 : hdlsllib/Sources/HDL Counter  CountType=Free running  CountInit=0  CountStep=1  CountMax=100  CountFromType=Initial value  CountFrom=0  CountResetPort=on  CountLoadPort=off  CountEnbPort=on  CountDirPort=off  CountHitOutputPort=off  CountDataType=Unsigned  CountWordLen=10  CountFracLen=0  CountSampTime=1
  n_perceptron : Outport
  write_enable : Outport  Port=2
  mac_counter : Outport  Port=3
  startin : Outport  Port=4
  endin : Outport  Port=5
  validIn : Outport  Port=6
  layer_rdy : Outport  Port=7
  layer_finished : Outport  Port=8
  wires:
  index_counter/1 -> Delay2/1, Scope/2, mac_counter/1  "mac_counter"
  end_out/1 -> mac_control/3(end_out), Delay3/1
  Relational Operator/1 -> layer_control/3(cnt_finished)
  mac_startOut/1 -> mac_control/5(mac_startOut)
  layer_control/5(layer_finished) -> layer_finished/1
  layer_control/2(layer_rdy) -> layer_rdy/1
  mac_control/6(write_ram) -> write_enable/1  "write_enable"
  Delay3/1 -> mac_control/4(end_out_delay)
  layer_control/3(cnt_enable) -> perceptron_counter1/2
  layer_control/1(enable_mac) -> mac_control/1(external_enable)
  mac_control/7(mac_ready) -> Delay4/1  "mac_ready"
  mac_control/2(mac_startIn) -> startin/1  "startin"
  Compare To Constant/1 -> mac_control/2(counter_finished)
  Delay2/1 -> Compare To Constant/1
  mac_control/1(index_counter_enb) -> index_counter/2
  Detect Rise Positive/1 -> layer_control/1(ext_enable)
  mac_control/5(index_counter_rst) -> index_counter/1
  mac_control/3(mac_endIn) -> endin/1  "endin"
  perceptron_counter1/1 -> Relational Operator/1, n_perceptron/1, Scope/1  "n_perceptron"
  layer_control/4(counter_rest) -> perceptron_counter1/1
  Delay4/1 -> layer_control/2(mac_ready)
  mac_control/4(mac_validIn) -> validIn/1  "validIn"
  U/1 -> Detect Rise Positive/1
  output_half_minus_one/1 -> Relational Operator/2

== system uz_mlp_three_layer/uz_mlp_three_layer/LastLayer/Subsystem1 ==
  mac_counter : Inport
  b : Inport  Port=2
  startin : Inport  Port=3
  endin : Inport  Port=4
  validIn : Inport  Port=5
  n_perceptron : Inport  Port=6
  axi_signals : Inport  Port=7
  AND : Logic  IconShape=distinctive  AllPortsSameDT=off  OutDataTypeStr=boolean
  AND1 : Logic  IconShape=distinctive  AllPortsSameDT=off  OutDataTypeStr=boolean
  Bus Selector : BusSelector  OutputSignals=axi_weightData,axi_weightAddr,axi_weightsWriteEnable,axi_biasData,axi_biasAddr,axi_biasWriteEnable,axi_layerNr
  Compare To Constant : simulink/Logic and Bit Operations/Compare To Constant  relop===  const=ParallelNr  OutDataTypeStr=boolean
  Compare To Constant1 : simulink/Logic and Bit Operations/Compare To Constant  relop===  const=ParallelNr  OutDataTypeStr=boolean
  Compare To Constant2 : simulink/Logic and Bit Operations/Compare To Constant  relop===  const=LayerNr  OutDataTypeStr=boolean
  Dual Port RAM System1 : hdlsllib/HDL RAMs/Dual Port RAM System  RAMType=Simple dual port  WriteOutputValue=New data  RAMInitialValue=[layer.bias(nStart:nEnd);zeros(1024-length(layer.bias(nStart:nEnd)),1)]  SimulateUsing=Code generation
      settings: SourceProductBaseCode=SL
  Dual Port RAM System3 : hdlsllib/HDL RAMs/Dual Port RAM System  RAMType=Simple dual port  WriteOutputValue=New data  RAMInitialValue=[0;reshape(layer.weights(:,nStart:nEnd),[],1);zeros(1023-length(reshape(layer.weights(:,nStart:nEnd),[],1)),1)]  SimulateUsing=Code generation
      settings: SourceProductBaseCode=SL
  Gain : Gain  Gain=size(layer.weights(:,nStart:nEnd),1)  OutDataTypeStr=Inherit: Same as input
  Multiply-Accumulate1 : hdlsllib/HDL Operations/Multiply-Accumulate  opMode=Streaming - using Start and End ports  initValueSetting=Dialog  initValue=0  initValueSetting2=Input port  initValue2=0  initValueSetting3=Dialog  initValue3=0  num_samples=2  RndMeth2=Floor  RndMeth3=Floor  datatype2=fixdt(1,32,14)  datatype3=Inherit: Inherit via back propagation  validOut=on  endInandOut=on  startOut=on  countOut=on  dim=-1  DoSatur=off  parallel=off
      settings: SourceProductBaseCode=SL
  Sum1 : Sum  Inputs=|++  OutDataTypeStr=Inherit: Same as first input
  Terminator : Terminator
  rd_dout : Outport
  startOut : Outport  Port=2
  endOut : Outport  Port=3
  wires:
  AND1/1 -> Dual Port RAM System1/3
  Bus Selector/7 -> Compare To Constant2/1  "<axi_layerNr>"
  AND/1 -> Dual Port RAM System3/3
  Compare To Constant2/1 -> AND/2, AND1/2
  Compare To Constant1/1 -> AND1/1
  Compare To Constant/1 -> AND/1
  axi_signals/1 -> Bus Selector/1
  Bus Selector/3 -> Compare To Constant/1  "<axi_weightsWriteEnable>"
  Bus Selector/2 -> Dual Port RAM System3/2  "<axi_weightAddr>"
  Bus Selector/1 -> Dual Port RAM System3/1  "<axi_weightData>"
  Bus Selector/6 -> Compare To Constant1/1  "<axi_biasWriteEnable>"
  Bus Selector/5 -> Dual Port RAM System1/2  "<axi_biasAddr>"
  Bus Selector/4 -> Dual Port RAM System1/1  "<axi_biasData>"
  Dual Port RAM System3/1 -> Multiply-Accumulate1/1
  Sum1/1 -> Dual Port RAM System3/4
  Gain/1 -> Sum1/1
  startin/1 -> Multiply-Accumulate1/3
  validIn/1 -> Multiply-Accumulate1/5
  mac_counter/1 -> Sum1/2
  Multiply-Accumulate1/3 -> endOut/1  "endout"
  endin/1 -> Multiply-Accumulate1/4
  n_perceptron/1 -> Gain/1, Dual Port RAM System1/4
  b/1 -> Multiply-Accumulate1/2
  Multiply-Accumulate1/1 -> rd_dout/1  "data"
  Multiply-Accumulate1/2 -> startOut/1  "startout"
  Multiply-Accumulate1/4 -> Terminator/1  "validout"
  Dual Port RAM System1/1 -> Multiply-Accumulate1/6  "c"

== system uz_mlp_three_layer/uz_mlp_three_layer/LastLayer/Subsystem8 ==
  mac_counter : Inport
  b : Inport  Port=2
  startin : Inport  Port=3
  endin : Inport  Port=4
  validIn : Inport  Port=5
  n_perceptron : Inport  Port=6
  axi_signals : Inport  Port=7
  AND : Logic  IconShape=distinctive  AllPortsSameDT=off  OutDataTypeStr=boolean
  AND1 : Logic  IconShape=distinctive  AllPortsSameDT=off  OutDataTypeStr=boolean
  Bus Selector : BusSelector  OutputSignals=axi_weightData,axi_weightAddr,axi_weightsWriteEnable,axi_biasData,axi_biasAddr,axi_biasWriteEnable,axi_layerNr
  Compare To Constant : simulink/Logic and Bit Operations/Compare To Constant  relop===  const=ParallelNr  OutDataTypeStr=boolean
  Compare To Constant1 : simulink/Logic and Bit Operations/Compare To Constant  relop===  const=ParallelNr  OutDataTypeStr=boolean
  Compare To Constant2 : simulink/Logic and Bit Operations/Compare To Constant  relop===  const=LayerNr  OutDataTypeStr=boolean
  Dual Port RAM System1 : hdlsllib/HDL RAMs/Dual Port RAM System  RAMType=Simple dual port  WriteOutputValue=New data  RAMInitialValue=[layer.bias(nStart:nEnd);zeros(1024-length(layer.bias(nStart:nEnd)),1)]  SimulateUsing=Code generation
      settings: SourceProductBaseCode=SL
  Dual Port RAM System3 : hdlsllib/HDL RAMs/Dual Port RAM System  RAMType=Simple dual port  WriteOutputValue=New data  RAMInitialValue=[0;reshape(layer.weights(:,nStart:nEnd),[],1);zeros(1023-length(reshape(layer.weights(:,nStart:nEnd),[],1)),1)]  SimulateUsing=Code generation
      settings: SourceProductBaseCode=SL
  Gain : Gain  Gain=size(layer.weights(:,nStart:nEnd),1)  OutDataTypeStr=Inherit: Same as input
  Multiply-Accumulate1 : hdlsllib/HDL Operations/Multiply-Accumulate  opMode=Streaming - using Start and End ports  initValueSetting=Dialog  initValue=0  initValueSetting2=Input port  initValue2=0  initValueSetting3=Dialog  initValue3=0  num_samples=2  RndMeth2=Floor  RndMeth3=Floor  datatype2=fixdt(1,32,14)  datatype3=Inherit: Inherit via back propagation  validOut=on  endInandOut=on  startOut=on  countOut=on  dim=-1  DoSatur=off  parallel=off
      settings: SourceProductBaseCode=SL
  Sum1 : Sum  Inputs=|++  OutDataTypeStr=Inherit: Same as first input
  Terminator : Terminator
  rd_dout : Outport
  startOut : Outport  Port=2
  endOut : Outport  Port=3
  wires:
  Dual Port RAM System1/1 -> Multiply-Accumulate1/6  "c"
  Multiply-Accumulate1/4 -> Terminator/1  "validout"
  Multiply-Accumulate1/2 -> startOut/1  "startout"
  Multiply-Accumulate1/1 -> rd_dout/1  "data"
  b/1 -> Multiply-Accumulate1/2
  n_perceptron/1 -> Dual Port RAM System1/4, Gain/1
  endin/1 -> Multiply-Accumulate1/4
  Multiply-Accumulate1/3 -> endOut/1  "endout"
  mac_counter/1 -> Sum1/2
  validIn/1 -> Multiply-Accumulate1/5
  startin/1 -> Multiply-Accumulate1/3
  Gain/1 -> Sum1/1
  Sum1/1 -> Dual Port RAM System3/4
  Dual Port RAM System3/1 -> Multiply-Accumulate1/1
  Bus Selector/4 -> Dual Port RAM System1/1  "<axi_biasData>"
  Bus Selector/5 -> Dual Port RAM System1/2  "<axi_biasAddr>"
  Bus Selector/6 -> Compare To Constant1/1  "<axi_biasWriteEnable>"
  Bus Selector/1 -> Dual Port RAM System3/1  "<axi_weightData>"
  Bus Selector/2 -> Dual Port RAM System3/2  "<axi_weightAddr>"
  Bus Selector/3 -> Compare To Constant/1  "<axi_weightsWriteEnable>"
  axi_signals/1 -> Bus Selector/1
  Compare To Constant/1 -> AND/1
  Compare To Constant1/1 -> AND1/1
  Compare To Constant2/1 -> AND1/2, AND/2
  AND/1 -> Dual Port RAM System3/3
  Bus Selector/7 -> Compare To Constant2/1  "<axi_layerNr>"
  AND1/1 -> Dual Port RAM System1/3

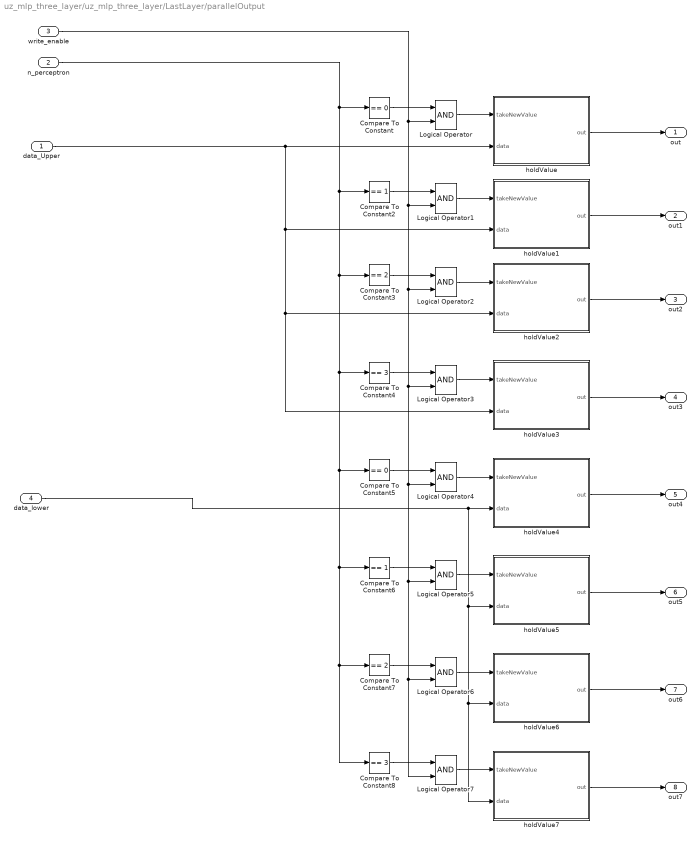
== system uz_mlp_three_layer/uz_mlp_three_layer/LastLayer/parallelOutput ==
  data_Upper : Inport
  n_perceptron : Inport  Port=2
  write_enable : Inport  Port=3
  data_lower : Inport  Port=4
  Compare To Constant : simulink/Logic and Bit Operations/Compare To Constant  relop===  const=0  OutDataTypeStr=boolean
  Compare To Constant2 : simulink/Logic and Bit Operations/Compare To Constant  relop===  const=1  OutDataTypeStr=boolean
  Compare To Constant3 : simulink/Logic and Bit Operations/Compare To Constant  relop===  const=2  OutDataTypeStr=boolean
  Compare To Constant4 : simulink/Logic and Bit Operations/Compare To Constant  relop===  const=3  OutDataTypeStr=boolean
  Compare To Constant5 : simulink/Logic and Bit Operations/Compare To Constant  relop===  const=0  OutDataTypeStr=boolean
  Compare To Constant6 : simulink/Logic and Bit Operations/Compare To Constant  relop===  const=1  OutDataTypeStr=boolean
  Compare To Constant7 : simulink/Logic and Bit Operations/Compare To Constant  relop===  const=2  OutDataTypeStr=boolean
  Compare To Constant8 : simulink/Logic and Bit Operations/Compare To Constant  relop===  const=3  OutDataTypeStr=boolean
  Logical Operator{,1..7} (8 alike) : Logic  AllPortsSameDT=off  OutDataTypeStr=boolean
  holdValue : Subsystem
  holdValue1 : Subsystem
  holdValue2 : Subsystem
  holdValue3 : Subsystem
  holdValue4 : Subsystem
  holdValue5 : Subsystem
  holdValue6 : Subsystem
  holdValue7 : Subsystem
  out : Outport
  out1 : Outport  Port=2
  out2 : Outport  Port=3
  out3 : Outport  Port=4
  out4 : Outport  Port=5
  out5 : Outport  Port=6
  out6 : Outport  Port=7
  out7 : Outport  Port=8
  wires:
  Compare To Constant2/1 -> Logical Operator1/1
  Logical Operator2/1 -> holdValue2/1(takeNewValue)
  Compare To Constant4/1 -> Logical Operator3/1
  Compare To Constant7/1 -> Logical Operator6/1
  Compare To Constant6/1 -> Logical Operator5/1
  Logical Operator7/1 -> holdValue7/1(takeNewValue)
  holdValue2/1(out) -> out2/1
  Logical Operator4/1 -> holdValue4/1(takeNewValue)
  holdValue/1(out) -> out/1
  Compare To Constant/1 -> Logical Operator/1
  holdValue1/1(out) -> out1/1
  holdValue4/1(out) -> out4/1
  write_enable/1 -> Logical Operator7/2, Logical Operator6/2, Logical Operator5/2, Logical Operator4/2, Logical Operator3/2, Logical Operator2/2, Logical Operator1/2, Logical Operator/2
  Logical Operator1/1 -> holdValue1/1(takeNewValue)
  Logical Operator5/1 -> holdValue5/1(takeNewValue)
  data_Upper/1 -> holdValue2/2(data), holdValue3/2(data), holdValue1/2(data), holdValue/2(data)
  holdValue3/1(out) -> out3/1
  holdValue7/1(out) -> out7/1
  Logical Operator/1 -> holdValue/1(takeNewValue)
  holdValue6/1(out) -> out6/1
  Compare To Constant3/1 -> Logical Operator2/1
  Compare To Constant5/1 -> Logical Operator4/1
  Compare To Constant8/1 -> Logical Operator7/1
  holdValue5/1(out) -> out5/1
  Logical Operator3/1 -> holdValue3/1(takeNewValue)
  n_perceptron/1 -> Compare To Constant8/1, Compare To Constant7/1, Compare To Constant6/1, Compare To Constant5/1, Compare To Constant4/1, Compare To Constant3/1, Compare To Constant2/1, Compare To Constant/1
  Logical Operator6/1 -> holdValue6/1(takeNewValue)
  data_lower/1 -> holdValue7/2(data), holdValue6/2(data), holdValue5/2(data), holdValue4/2(data)

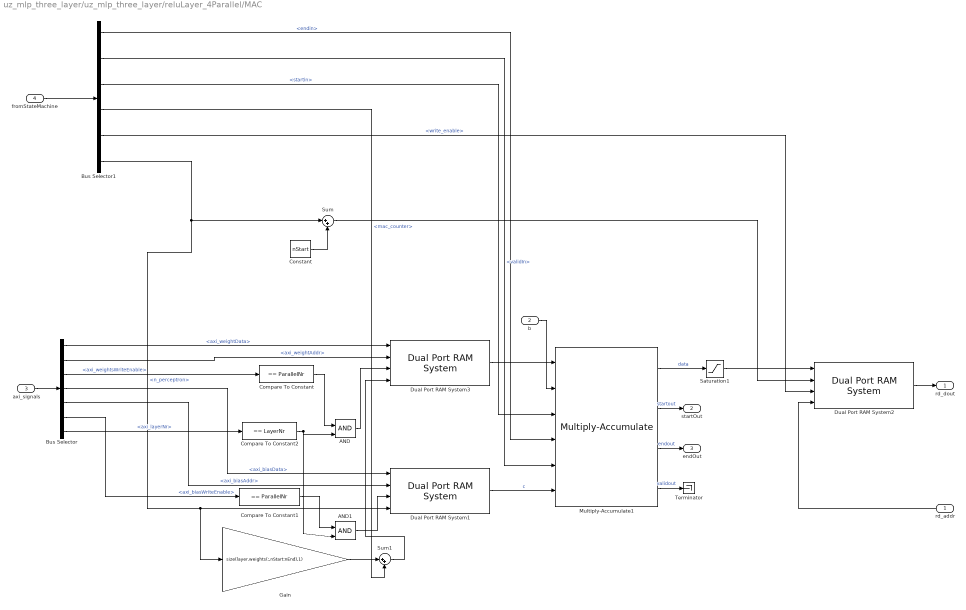
== system uz_mlp_three_layer/uz_mlp_three_layer/reluLayer_4Parallel/MAC ==
  rd_addr : Inport
  b : Inport  Port=2
  axi_signals : Inport  Port=3
  fromStateMachine : Inport  Port=4
  AND : Logic  IconShape=distinctive  AllPortsSameDT=off  OutDataTypeStr=boolean
  AND1 : Logic  IconShape=distinctive  AllPortsSameDT=off  OutDataTypeStr=boolean
  Bus Selector : BusSelector  OutputSignals=axi_weightData,axi_weightAddr,axi_weightsWriteEnable,axi_biasData,axi_biasAddr,axi_biasWriteEnable,axi_layerNr
  Bus Selector1 : BusSelector  OutputSignals=endin,validIn,startin,mac_counter,write_enable,n_perceptron
  Compare To Constant : simulink/Logic and Bit Operations/Compare To Constant  relop===  const=ParallelNr  OutDataTypeStr=boolean
  Compare To Constant1 : simulink/Logic and Bit Operations/Compare To Constant  relop===  const=ParallelNr  OutDataTypeStr=boolean
  Compare To Constant2 : simulink/Logic and Bit Operations/Compare To Constant  relop===  const=LayerNr  OutDataTypeStr=boolean
  Constant : Constant  Value=nStart  OutDataTypeStr=Inherit: Inherit via back propagation  SampleTime=-1
  Dual Port RAM System1 : hdlsllib/HDL RAMs/Dual Port RAM System  RAMType=Simple dual port  WriteOutputValue=New data  RAMInitialValue=[layer.bias(nStart:nEnd);zeros(1024-length(layer.bias(nStart:nEnd)),1)]  SimulateUsing=Code generation
      settings: SourceProductBaseCode=SL
  Dual Port RAM System2 : hdlsllib/HDL RAMs/Dual Port RAM System  RAMType=Simple dual port  WriteOutputValue=New data  RAMInitialValue=[0]  SimulateUsing=Code generation
      settings: SourceProductBaseCode=SL
  Dual Port RAM System3 : hdlsllib/HDL RAMs/Dual Port RAM System  RAMType=Simple dual port  WriteOutputValue=New data  RAMInitialValue=[0;reshape(layer.weights(:,nStart:nEnd),[],1);zeros(1023-length(reshape(layer.weights(:,nStart:nEnd),[],1)),1)]  SimulateUsing=Code generation
      settings: SourceProductBaseCode=SL
  Gain : Gain  Gain=size(layer.weights(:,nStart:nEnd),1)  OutDataTypeStr=Inherit: Same as input
  Multiply-Accumulate1 : hdlsllib/HDL Operations/Multiply-Accumulate  opMode=Streaming - using Start and End ports  initValueSetting=Dialog  initValue=0  initValueSetting2=Input port  initValue2=0  initValueSetting3=Dialog  initValue3=0  num_samples=2  RndMeth2=Floor  RndMeth3=Floor  datatype2=fixdt(1,32,14)  datatype3=Inherit: Inherit via back propagation  validOut=on  endInandOut=on  startOut=on  countOut=on  dim=-1  DoSatur=off  parallel=off
      settings: SourceProductBaseCode=SL
  Saturation1 : Saturate  UpperLimit=nn_data_type_max  LowerLimit=0
  Sum : Sum  Inputs=|++  OutDataTypeStr=Inherit: Same as first input
  Sum1 : Sum  Inputs=|++  OutDataTypeStr=Inherit: Same as first input
  Terminator : Terminator
  rd_dout : Outport
  startOut : Outport  Port=2
  endOut : Outport  Port=3
  wires:
  Dual Port RAM System1/1 -> Multiply-Accumulate1/6  "c"
  Saturation1/1 -> Dual Port RAM System2/1
  Multiply-Accumulate1/4 -> Terminator/1  "validout"
  Multiply-Accumulate1/2 -> startOut/1  "startout"
  Multiply-Accumulate1/1 -> Saturation1/1  "data"
  b/1 -> Multiply-Accumulate1/2
  Bus Selector1/6 -> Sum/1, Dual Port RAM System1/4, Gain/1  "<n_perceptron>"
  Constant/1 -> Sum/2
  Bus Selector1/1 -> Multiply-Accumulate1/4  "<endin>"
  Multiply-Accumulate1/3 -> endOut/1  "endout"
  Dual Port RAM System2/1 -> rd_dout/1
  Bus Selector1/4 -> Sum1/2  "<mac_counter>"
  Bus Selector1/2 -> Multiply-Accumulate1/5  "<validIn>"
  Bus Selector1/3 -> Multiply-Accumulate1/3  "<startin>"
  Gain/1 -> Sum1/1
  Sum1/1 -> Dual Port RAM System3/4
  Sum/1 -> Dual Port RAM System2/2
  Bus Selector1/5 -> Dual Port RAM System2/3  "<write_enable>"
  rd_addr/1 -> Dual Port RAM System2/4
  Dual Port RAM System3/1 -> Multiply-Accumulate1/1
  Bus Selector/4 -> Dual Port RAM System1/1  "<axi_biasData>"
  Bus Selector/5 -> Dual Port RAM System1/2  "<axi_biasAddr>"
  Bus Selector/6 -> Compare To Constant1/1  "<axi_biasWriteEnable>"
  Bus Selector/1 -> Dual Port RAM System3/1  "<axi_weightData>"
  Bus Selector/2 -> Dual Port RAM System3/2  "<axi_weightAddr>"
  Bus Selector/3 -> Compare To Constant/1  "<axi_weightsWriteEnable>"
  axi_signals/1 -> Bus Selector/1
  Compare To Constant/1 -> AND/1
  Compare To Constant1/1 -> AND1/1
  Compare To Constant2/1 -> AND1/2, AND/2
  AND/1 -> Dual Port RAM System3/3
  Bus Selector/7 -> Compare To Constant2/1  "<axi_layerNr>"
  AND1/1 -> Dual Port RAM System1/3
  fromStateMachine/1 -> Bus Selector1/1
